simulink model "untitled"  (R2014a)
settings: Solver=ode45  StartTime=0.0  StopTime=10.0  RelTol=1e-3
settings Model: Creator=SKY  LastModifiedBy=SKY

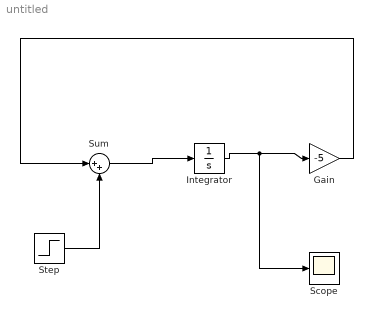
== system untitled ==
  Gain : Gain  Gain=-5
  Integrator : Integrator  InitialCondition=-2
  Scope : Scope
  Step : Step  SampleTime=0
  Sum : Sum  Inputs=|++
  wires:
  Integrator/1 -> Scope/1, Gain/1
  Sum/1 -> Integrator/1
  Step/1 -> Sum/2
  Gain/1 -> Sum/1
